simulink subsystem "PvtSubSys_AHBC"  (R2020b)
settings: Solver=VariableStepAuto  StartTime=0.0  StopTime=10.0  RelTol=1e-3
undefined symbols (not defined in the file): P_AHBC_ABS_ENABLE, P_AHBC_DRIVE_DIRECTION_ENABLE, P_AHBC_ESP_ENABLE, P_AHBC_FOG_ENABLE, P_AHBC_FOG_TIME, P_AHBC_HIGHBEAM_ACTIVE_GRACE, P_AHBC_LAT_ACC_ENTER, P_AHBC_LAT_ACC_EXIT, P_AHBC_MAX_ONCOMING_DISTANCE_COUPLE2, P_AHBC_MAX_ONCOMING_DISTANCE_ONE2, P_AHBC_MAX_TAILLIGHT_DISTANCE_COUPLE2, P_AHBC_MAX_TAILLIGHT_DISTANCE_ONE2, P_AHBC_SPEED_SWITCH_HIGH_BEAM_OFF2, P_AHBC_SPEED_SWITCH_HIGH_BEAM_ON2, P_AHBC_TrafficStyle, P_AHBC_TURN_LAMP_ENABLE, P_AHBC_WIPER_ENABLE, P_AHBC_WIPER_TIME, P_AHBC_YAW_RATE_ENTER, P_AHBC_YAW_RATE_EXIT
libraries: simulink x57
(part 2 of 4)

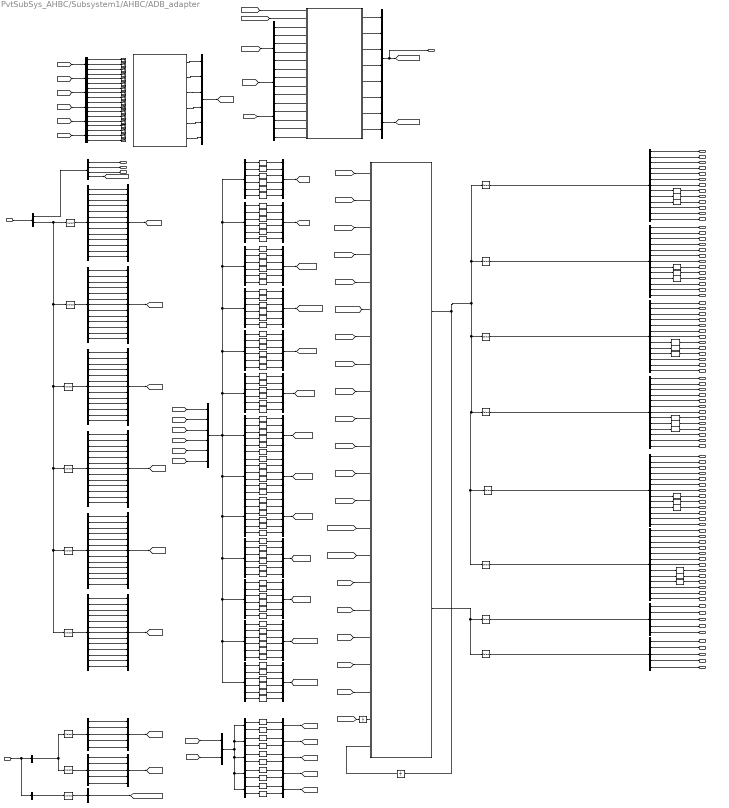
== system PvtSubSys_AHBC/Subsystem1/AHBC/ADB_adapter ==
  EQ4_LSV : Inport  OutDataTypeStr=Bus: EQ4_LSV_BUS
  EQ4_LSR : Inport  Port=2  OutDataTypeStr=Bus: EQ4_LSR_BUS
  Bus Creator{,1..5} (6 alike) : BusCreator  Inputs=13
  Bus Creator{6..20,30} (16 alike) : BusCreator  Inputs=6
  Bus Creator21 : BusCreator  Inputs=5
  Bus Creator22 : BusCreator  Inputs=5
  Bus Creator{23..29} (7 alike) : BusCreator  Inputs=2
  Bus Selector : BusSelector  OutputSignals=EQ4_LSV_HDR,EQ4_LSV_ELEM
  Bus Selector{1..6} (6 alike) : BusSelector  OutputSignals=LSV_ID,LSV_Is_New,LSV_Confidence,LSV_Consecutive_Detection,LSV_Type,LSV_Sub_Type,LSV_CL_Sub_Type,LSV_Distance,LSV_Right_Angle,LSV_Left_Angle,LSV_Top_Angle,LSV_Angular_Velocity_Right,LSV_Angular_Velocity_Left
  Bus Selector10 : BusSelector  OutputSignals=LSV_Running_Mode,LSV_HLB_Decision,LSV_HLB_Reason,LSV_Vehicles_Count
  Bus Selector11 : BusSelector  OutputSignals=EQ4_LSR_HDR
  Bus Selector12 : BusSelector  OutputSignals=LSR_Strong_Reflectors_Count
  Bus Selector13 : BusSelector  OutputSignals=LSV_Elem1.LSV_ID,LSV_Elem2.LSV_ID,LSV_Elem3.LSV_ID,LSV_Elem4.LSV_ID,LSV_Elem5.LSV_ID,LSV_Elem6.LSV_ID
  Bus Selector14 : BusSelector  OutputSignals=LSV_Elem1.LSV_Is_New,LSV_Elem2.LSV_Is_New,LSV_Elem3.LSV_Is_New,LSV_Elem4.LSV_Is_New,LSV_Elem5.LSV_Is_New,LSV_Elem6.LSV_Is_New
  Bus Selector15 : BusSelector  OutputSignals=LSV_Elem1.LSV_Confidence,LSV_Elem2.LSV_Confidence,LSV_Elem3.LSV_Confidence,LSV_Elem4.LSV_Confidence,LSV_Elem5.LSV_Confidence,LSV_Elem6.LSV_Confidence
  Bus Selector16 : BusSelector  OutputSignals=LSV_Elem1.LSV_Consecutive_Detection,LSV_Elem2.LSV_Consecutive_Detection,LSV_Elem3.LSV_Consecutive_Detection,LSV_Elem4.LSV_Consecutive_Detection,LSV_Elem5.LSV_Consecutive_Detection,LSV_Elem6.LSV_Consecutive_Detection
  Bus Selector17 : BusSelector  OutputSignals=LSV_Elem1.LSV_Type,LSV_Elem2.LSV_Type,LSV_Elem3.LSV_Type,LSV_Elem4.LSV_Type,LSV_Elem5.LSV_Type,LSV_Elem6.LSV_Type
  Bus Selector18 : BusSelector  OutputSignals=LSV_Elem1.LSV_Sub_Type,LSV_Elem2.LSV_Sub_Type,LSV_Elem3.LSV_Sub_Type,LSV_Elem4.LSV_Sub_Type,LSV_Elem5.LSV_Sub_Type,LSV_Elem6.LSV_Sub_Type
  Bus Selector19 : BusSelector  OutputSignals=LSV_Elem1.LSV_CL_Sub_Type,LSV_Elem2.LSV_CL_Sub_Type,LSV_Elem3.LSV_CL_Sub_Type,LSV_Elem4.LSV_CL_Sub_Type,LSV_Elem5.LSV_CL_Sub_Type,LSV_Elem6.LSV_CL_Sub_Type
  Bus Selector20 : BusSelector  OutputSignals=LSV_Elem1.LSV_Distance,LSV_Elem2.LSV_Distance,LSV_Elem3.LSV_Distance,LSV_Elem4.LSV_Distance,LSV_Elem5.LSV_Distance,LSV_Elem6.LSV_Distance
  Bus Selector21 : BusSelector  OutputSignals=LSV_Elem1.LSV_Right_Angle,LSV_Elem2.LSV_Right_Angle,LSV_Elem3.LSV_Right_Angle,LSV_Elem4.LSV_Right_Angle,LSV_Elem5.LSV_Right_Angle,LSV_Elem6.LSV_Right_Angle
  Bus Selector22 : BusSelector  OutputSignals=LSV_Elem1.LSV_Left_Angle,LSV_Elem2.LSV_Left_Angle,LSV_Elem3.LSV_Left_Angle,LSV_Elem4.LSV_Left_Angle,LSV_Elem5.LSV_Left_Angle,LSV_Elem6.LSV_Left_Angle
  Bus Selector23 : BusSelector  OutputSignals=LSV_Elem1.LSV_Top_Angle,LSV_Elem2.LSV_Top_Angle,LSV_Elem3.LSV_Top_Angle,LSV_Elem4.LSV_Top_Angle,LSV_Elem5.LSV_Top_Angle,LSV_Elem6.LSV_Top_Angle
  Bus Selector24 : BusSelector  OutputSignals=LSV_Elem1.LSV_Angular_Velocity_Right,LSV_Elem2.LSV_Angular_Velocity_Right,LSV_Elem3.LSV_Angular_Velocity_Right,LSV_Elem4.LSV_Angular_Velocity_Right,LSV_Elem5.LSV_Angular_Velocity_Right,LSV_Elem6.LSV_Angular_Velocity_Right
  Bus Selector25 : BusSelector  OutputSignals=LSV_Elem1.LSV_Angular_Velocity_Left,LSV_Elem2.LSV_Angular_Velocity_Left,LSV_Elem3.LSV_Angular_Velocity_Left,LSV_Elem4.LSV_Angular_Velocity_Left,LSV_Elem5.LSV_Angular_Velocity_Left,LSV_Elem6.LSV_Angular_Velocity_Left
  Bus Selector{26,28..32} (6 alike) : BusSelector  OutputSignals=LSV_ID_Out,LSV_Is_New_Out,LSV_Confidence_Out,LSV_Consecutive_Detection_Out,LSV_Type_Out,LSV_Sub_Type_Out,LSV_CL_Sub_Type_Out,LSV_Distance_Out,LSV_Right_Angle_Out,LSV_Left_Angle_Out,LSV_Top_Angle_Out,LSV_Angular_Velocity_Right_Out,LSV_Angular_Velocity_Left_Out
  Bus Selector27 : BusSelector  OutputSignals=LSV_Distance1,LSV_Distance2,LSV_Distance3,LSV_Distance4,LSV_Distance5,LSV_Distance6
  Bus Selector33 : BusSelector  OutputSignals=LSR_Elem1.LSR_ID,LSR_Elem2.LSR_ID
  Bus Selector34 : BusSelector  OutputSignals=LSR_Elem1.LSR_Distance,LSR_Elem2.LSR_Distance
  Bus Selector35 : BusSelector  OutputSignals=LSR_Elem1.LSR_Right_Angle,LSR_Elem2.LSR_Right_Angle
  Bus Selector36 : BusSelector  OutputSignals=LSR_Elem1.LSR_Left_Angle,LSR_Elem2.LSR_Left_Angle
  Bus Selector37 : BusSelector  OutputSignals=LSR_Elem1.LSR_Top_Angle,LSR_Elem2.LSR_Top_Angle
  Bus Selector38 : BusSelector  OutputSignals=LSR_Distance1,LSR_Distance2
  Bus Selector39 : BusSelector  OutputSignals=LSR_ID_Out,LSR_Distance_Out,LSR_Right_Angle_Out,LSR_Left_Angle_Out,LSR_Top_Angle_Out
  Bus Selector40 : BusSelector  OutputSignals=LSR_ID_Out,LSR_Distance_Out,LSR_Right_Angle_Out,LSR_Left_Angle_Out,LSR_Top_Angle_Out
  Bus Selector{41..46} (6 alike) : BusSelector  OutputSignals=LSV_Left_Angle,LSV_Right_Angle,LSV_Distance
  Bus Selector47 : BusSelector  OutputSignals=Target1_valid,Target2_valid,Target3_valid,Target4_valid,Target5_valid,Target6_valid
  Bus Selector7 : BusSelector  OutputSignals=EQ4_LSR_ELEM
  Bus Selector8 : BusSelector  OutputSignals=LSR_ID,LSR_Distance,LSR_Right_Angle,LSR_Left_Angle,LSR_Top_Angle
  Bus Selector9 : BusSelector  OutputSignals=LSR_ID,LSR_Distance,LSR_Right_Angle,LSR_Left_Angle,LSR_Top_Angle
  MATLAB Function : MATLAB Function  TreatAsAtomicUnit=on
  MATLAB Function1 : MATLAB Function  TreatAsAtomicUnit=on
  MATLAB Function2 : MATLAB Function  TreatAsAtomicUnit=on
  Selector : Selector  InputPortWidth=2  IndexOptions=Index vector (dialog)  Indices=1  OutputSizes=1
  Selector1 : Selector  InputPortWidth=2  IndexOptions=Index vector (dialog)  Indices=2  OutputSizes=1
  Selector10 : Selector  InputPortWidth=2  IndexOptions=Index vector (dialog)  Indices=1  OutputSizes=1
  Selector11 : Selector  InputPortWidth=2  IndexOptions=Index vector (dialog)  Indices=2  OutputSizes=1
  Selector14 : Selector  InputPortWidth=6  IndexOptions=Index vector (dialog)  Indices=2  OutputSizes=1
  Selector15 : Selector  InputPortWidth=6  IndexOptions=Index vector (dialog)  Indices=6  OutputSizes=1
  Selector16 : Selector  InputPortWidth=6  IndexOptions=Index vector (dialog)  Indices=3  OutputSizes=1
  Selector2 : Selector  InputPortWidth=6  IndexOptions=Index vector (dialog)  Indices=1  OutputSizes=1
  Selector23 : Selector  InputPortWidth=6  IndexOptions=Index vector (dialog)  Indices=5  OutputSizes=1
  Selector3 : Selector  InputPortWidth=1  IndexOptions=Index vector (dialog)  Indices=1  OutputSizes=1
  Selector30 : Selector  InputPortWidth=6  IndexOptions=Index vector (dialog)  Indices=4  OutputSizes=1
  Selector4 : Selector  InputPortWidth=6  IndexOptions=Index vector (dialog)  Indices=1  OutputSizes=1
  Selector5 : Selector  InputPortWidth=6  IndexOptions=Index vector (dialog)  Indices=2  OutputSizes=1
  Selector6 : Selector  InputPortWidth=6  IndexOptions=Index vector (dialog)  Indices=3  OutputSizes=1
  Selector7 : Selector  InputPortWidth=6  IndexOptions=Index vector (dialog)  Indices=4  OutputSizes=1
  Selector8 : Selector  InputPortWidth=6  IndexOptions=Index vector (dialog)  Indices=5  OutputSizes=1
  Selector9 : Selector  InputPortWidth=6  IndexOptions=Index vector (dialog)  Indices=6  OutputSizes=1
  Signal Conversion{,1..105} (106 alike) : SignalConversion  OverrideOpt=off
  Terminator{,1..17} (18 alike) : Terminator
  Unit Delay : UnitDelay  SampleTime=-1  HasFrameUpgradeWarning=on
  Unit Delay1 : UnitDelay  SampleTime=-1  HasFrameUpgradeWarning=on
  LSV_Running_Mode : Outport
  LSV_HLB_Decision : Outport  Port=2
  LSV_HLB_Reason : Outport  Port=3
  LSV_ID1 : Outport  Port=4
  LSV_Is_New1 : Outport  Port=5
  LSV_Confidence1 : Outport  Port=6
  LSV_Consecutive_Detection1 : Outport  Port=7
  LSV_Type1 : Outport  Port=8
  LSV_Sub_Type1 : Outport  Port=9
  LSV_CL_Sub_Type1 : Outport  Port=10
  LSV_Distance1 : Outport  Port=11  OutDataTypeStr=uint16
  LSV_Right_Angle1 : Outport  Port=12
  LSV_Left_Angle1 : Outport  Port=13
  LSV_Top_Angle1 : Outport  Port=14
  LSV_Angular_Velocity_Right1 : Outport  Port=15
  LSV_Angular_Velocity_Left1 : Outport  Port=16
  LSV_ID2 : Outport  Port=17
  LSV_Is_New2 : Outport  Port=18
  LSV_Confidence2 : Outport  Port=19
  LSV_Consecutive_Detection2 : Outport  Port=20
  LSV_Type2 : Outport  Port=21
  LSV_Distance2 : Outport  Port=22  OutDataTypeStr=uint16
  LSV_Right_Angle2 : Outport  Port=23
  LSV_Left_Angle2 : Outport  Port=24
  LSV_Top_Angle2 : Outport  Port=25
  LSV_Angular_Velocity_Right2 : Outport  Port=26
  LSV_Angular_Velocity_Left2 : Outport  Port=27
  LSV_Sub_Type2 : Outport  Port=28
  LSV_CL_Sub_Type2 : Outport  Port=29
  LSV_ID3 : Outport  Port=30
  LSV_Is_New3 : Outport  Port=31
  LSV_Confidence3 : Outport  Port=32
  LSV_Consecutive_Detection3 : Outport  Port=33
  LSV_Type3 : Outport  Port=34
  LSV_Sub_Type3 : Outport  Port=35
  LSV_CL_Sub_Type3 : Outport  Port=36
  LSV_Distance3 : Outport  Port=37  OutDataTypeStr=uint16
  LSV_Right_Angle3 : Outport  Port=38
  LSV_Left_Angle3 : Outport  Port=39
  LSV_Top_Angle3 : Outport  Port=40
  LSV_Angular_Velocity_Right3 : Outport  Port=41
  LSV_Angular_Velocity_Left3 : Outport  Port=42
  LSV_ID4 : Outport  Port=43
  LSV_Is_New4 : Outport  Port=44
  LSV_Confidence4 : Outport  Port=45
  LSV_Consecutive_Detection4 : Outport  Port=46
  LSV_Type4 : Outport  Port=47
  LSV_Sub_Type4 : Outport  Port=48
  LSV_CL_Sub_Type4 : Outport  Port=49
  LSV_Distance4 : Outport  Port=50  OutDataTypeStr=uint16
  LSV_Right_Angle4 : Outport  Port=51
  LSV_Left_Angle4 : Outport  Port=52
  LSV_Top_Angle4 : Outport  Port=53
  LSV_Angular_Velocity_Right4 : Outport  Port=54
  LSV_Angular_Velocity_Left4 : Outport  Port=55
  LSV_ID5 : Outport  Port=56
  LSV_Is_New5 : Outport  Port=57
  LSV_Confidence5 : Outport  Port=58
  LSV_Consecutive_Detection5 : Outport  Port=59
  LSV_Type5 : Outport  Port=60
  LSV_Sub_Type5 : Outport  Port=61
  LSV_CL_Sub_Type5 : Outport  Port=62
  LSV_Distance5 : Outport  Port=63  OutDataTypeStr=uint16
  LSV_Right_Angle5 : Outport  Port=64
  LSV_Left_Angle5 : Outport  Port=65
  LSV_Top_Angle5 : Outport  Port=66
  LSV_Angular_Velocity_Right5 : Outport  Port=67
  LSV_Angular_Velocity_Left5 : Outport  Port=68
  LSV_ID6 : Outport  Port=69
  LSV_Is_New6 : Outport  Port=70
  LSV_Confidence6 : Outport  Port=71
  LSV_Consecutive_Detection6 : Outport  Port=72
  LSV_Type6 : Outport  Port=73
  LSV_Sub_Type6 : Outport  Port=74
  LSV_CL_Sub_Type6 : Outport  Port=75
  LSV_Distance6 : Outport  Port=76  OutDataTypeStr=uint16
  LSV_Right_Angle6 : Outport  Port=77
  LSV_Left_Angle6 : Outport  Port=78
  LSV_Top_Angle6 : Outport  Port=79
  LSV_Angular_Velocity_Right6 : Outport  Port=80
  LSV_Angular_Velocity_Left6 : Outport  Port=81
  LSR_ID1 : Outport  Port=82
  LSR_Distance1 : Outport  Port=83  OutDataTypeStr=uint16
  LSR_Right_Angle1 : Outport  Port=84
  LSR_Left_Angle1 : Outport  Port=85
  LSR_Top_Angle1 : Outport  Port=86
  LSR_ID2 : Outport  Port=87
  LSR_Distance2 : Outport  Port=88  OutDataTypeStr=uint16
  LSR_Right_Angle2 : Outport  Port=89
  LSR_Left_Angle2 : Outport  Port=90
  LSR_Top_Angle2 : Outport  Port=91
  LSV_valid_state : Outport  Port=92
  wires:
  Bus Selector46/3 -> Terminator16/1  "<LSV_Distance>"
  Bus Selector46/2 -> Terminator15/1  "<LSV_Right_Angle>"
  Bus Selector46/1 -> Terminator17/1  "<LSV_Left_Angle>"
  Bus Selector45/1 -> Terminator14/1  "<LSV_Left_Angle>"
  Bus Selector45/2 -> Terminator12/1  "<LSV_Right_Angle>"
  Bus Selector45/3 -> Terminator13/1  "<LSV_Distance>"
  Bus Selector44/3 -> Terminator11/1  "<LSV_Distance>"
  Bus Selector44/2 -> Terminator10/1  "<LSV_Right_Angle>"
  Bus Selector44/1 -> Terminator9/1  "<LSV_Left_Angle>"
  Bus Selector43/3 -> Terminator8/1  "<LSV_Distance>"
  Bus Selector43/2 -> Terminator7/1  "<LSV_Right_Angle>"
  Bus Selector43/1 -> Terminator6/1  "<LSV_Left_Angle>"
  Bus Selector42/3 -> Terminator5/1  "<LSV_Distance>"
  Bus Selector42/2 -> Terminator4/1  "<LSV_Right_Angle>"
  Bus Selector42/1 -> Terminator3/1  "<LSV_Left_Angle>"
  Bus Selector41/3 -> Terminator2/1  "<LSV_Distance>"
  Bus Selector41/2 -> Terminator1/1  "<LSV_Right_Angle>"
  Bus Selector41/1 -> Terminator/1  "<LSV_Left_Angle>"
  Unit Delay1/1 -> MATLAB Function1/21(LSV_valid_stateK)
  [LSV_valid_state] -> Unit Delay1/1
  Bus Creator30/1 -> [Target_valid]
  MATLAB Function2/6(Target6_valid) -> Bus Creator30/6
  MATLAB Function2/5(Target5_valid) -> Bus Creator30/5
  MATLAB Function2/4(Target4_valid) -> Bus Creator30/4
  MATLAB Function2/3(Target3_valid) -> Bus Creator30/3
  MATLAB Function2/2(Target2_valid) -> Bus Creator30/2
  MATLAB Function2/1(Target1_valid) -> Bus Creator30/1
  [LSV_Elem6] -> Bus Selector46/1
  [LSV_Elem5] -> Bus Selector45/1
  [LSV_Elem4] -> Bus Selector44/1
  [LSV_Elem3] -> Bus Selector43/1
  [LSV_Elem2] -> Bus Selector42/1
  Signal Conversion14/1 -> LSV_Right_Angle6/1
  Signal Conversion15/1 -> LSV_Left_Angle6/1
  Signal Conversion13/1 -> LSV_Distance6/1
  Signal Conversion104/1 -> LSV_Right_Angle5/1
  Signal Conversion103/1 -> LSV_Distance5/1
  Signal Conversion105/1 -> LSV_Left_Angle5/1
  Signal Conversion101/1 -> LSV_Right_Angle4/1
  Signal Conversion102/1 -> LSV_Left_Angle4/1
  Signal Conversion100/1 -> LSV_Distance4/1
  Signal Conversion99/1 -> LSV_Left_Angle3/1
  Signal Conversion97/1 -> LSV_Distance3/1
  Signal Conversion98/1 -> LSV_Right_Angle3/1
  Signal Conversion16/1 -> LSV_Distance2/1
  Signal Conversion17/1 -> LSV_Right_Angle2/1
  Signal Conversion96/1 -> LSV_Left_Angle2/1
  Signal Conversion12/1 -> LSV_Left_Angle1/1
  Signal Conversion11/1 -> LSV_Right_Angle1/1
  Signal Conversion/1 -> LSV_Distance1/1
  Selector11/1 -> Bus Selector40/1
  Selector10/1 -> Bus Selector39/1
  Bus Selector40/5 -> LSR_Top_Angle2/1  "<LSR_Top_Angle_Out>"
  Bus Selector40/4 -> LSR_Left_Angle2/1  "<LSR_Left_Angle_Out>"
  Bus Selector40/3 -> LSR_Right_Angle2/1  "<LSR_Right_Angle_Out>"
  Bus Selector40/2 -> LSR_Distance2/1  "<LSR_Distance_Out>"
  Bus Selector40/1 -> LSR_ID2/1  "<LSR_ID_Out>"
  Bus Selector39/5 -> LSR_Top_Angle1/1  "<LSR_Top_Angle_Out>"
  Bus Selector39/4 -> LSR_Left_Angle1/1  "<LSR_Left_Angle_Out>"
  Bus Selector39/3 -> LSR_Right_Angle1/1  "<LSR_Right_Angle_Out>"
  Bus Selector39/2 -> LSR_Distance1/1  "<LSR_Distance_Out>"
  Bus Selector39/1 -> LSR_ID1/1  "<LSR_ID_Out>"
  MATLAB Function1/2(LSR_List) -> Selector11/1, Selector10/1
  [LSR_Left_Angle] -> MATLAB Function1/19(LSR_Left_Angle)
  [LSR_Top_Angle] -> MATLAB Function1/20(LSR_Top_Angle)
  [LSR_Right_Angle] -> MATLAB Function1/18(LSR_Right_Angle)
  [LSR_Distance] -> MATLAB Function1/17(LSR_Distance)
  [LSR_ID] -> MATLAB Function1/16(LSR_ID)
  [LSR_valid_state] -> MATLAB Function1/2(LSR_valid_state)
  Bus Creator29/1 -> [LSR_valid_state]  "LSR_valid_state"
  MATLAB Function/7(LSR_valid_state1) -> Bus Creator29/1
  MATLAB Function/8(LSR_valid_state2) -> Bus Creator29/2
  MATLAB Function/6(LSV_valid_state6) -> Bus Creator20/6
  MATLAB Function/5(LSV_valid_state5) -> Bus Creator20/5
  MATLAB Function/4(LSV_valid_state4) -> Bus Creator20/4
  MATLAB Function/3(LSV_valid_state3) -> Bus Creator20/3
  MATLAB Function/2(LSV_valid_state2) -> Bus Creator20/2
  MATLAB Function/1(LSV_valid_state1) -> Bus Creator20/1
  Bus Selector38/2 -> MATLAB Function/10(LSR_Distance2)  "<LSR_Distance2>"
  Bus Selector38/1 -> MATLAB Function/9(LSR_Distance1)  "<LSR_Distance1>"
  [LSR_Distance] -> Bus Selector38/1
  Bus Creator28/1 -> [LSR_Top_Angle]  "LSR_Top_Angle"
  Bus Creator27/1 -> [LSR_Left_Angle]  "LSR_Left_Angle"
  Bus Creator26/1 -> [LSR_Right_Angle]  "LSR_Right_Angle"
  Bus Creator25/1 -> [LSR_Distance]  "LSR_Distance"
  Bus Creator24/1 -> [LSR_ID]  "LSR_ID"
  Signal Conversion10/1 -> Bus Creator28/2  "LSR_Top_Angle2"
  Signal Conversion9/1 -> Bus Creator28/1  "LSR_Top_Angle1"
  Signal Conversion8/1 -> Bus Creator27/2  "LSR_Left_Angle2"
  Signal Conversion7/1 -> Bus Creator27/1  "LSR_Left_Angle1"
  Signal Conversion6/1 -> Bus Creator26/2  "LSR_Right_Angle2"
  Signal Conversion5/1 -> Bus Creator26/1  "LSR_Right_Angle1"
  Signal Conversion4/1 -> Bus Creator25/2  "LSR_Distance2"
  Signal Conversion3/1 -> Bus Creator25/1  "LSR_Distance1"
  Signal Conversion2/1 -> Bus Creator24/2  "LSR_ID2"
  Signal Conversion1/1 -> Bus Creator24/1  "LSR_ID1"
  Bus Selector37/2 -> Signal Conversion10/1  "<LSR_Top_Angle>"
  Bus Selector37/1 -> Signal Conversion9/1  "<LSR_Top_Angle>"
  Bus Selector36/2 -> Signal Conversion8/1  "<LSR_Left_Angle>"
  Bus Selector36/1 -> Signal Conversion7/1  "<LSR_Left_Angle>"
  Bus Selector35/2 -> Signal Conversion6/1  "<LSR_Right_Angle>"
  Bus Selector35/1 -> Signal Conversion5/1  "<LSR_Right_Angle>"
  Bus Selector34/2 -> Signal Conversion4/1  "<LSR_Distance>"
  Bus Selector34/1 -> Signal Conversion3/1  "<LSR_Distance>"
  Bus Selector33/2 -> Signal Conversion2/1  "<LSR_ID>"
  Bus Selector33/1 -> Signal Conversion1/1  "<LSR_ID>"
  Bus Creator23/1 -> Bus Selector35/1, Bus Selector36/1, Bus Selector37/1, Bus Selector33/1, Bus Selector34/1
  [LSR_Elem2] -> Bus Creator23/2
  [LSR_Elem1] -> Bus Creator23/1
  Bus Creator22/1 -> [LSR_Elem2]  "LSR_Elem2"
  Bus Creator21/1 -> [LSR_Elem1]  "LSR_Elem1"
  [LSR_Strong_Reflectors_Count] -> MATLAB Function/2(LSR_Strong_Reflectors_Count)
  Bus Selector12/1 -> [LSR_Strong_Reflectors_Count]  "<LSR_Strong_Reflectors_Count>"
  Bus Selector8/5 -> Bus Creator22/5  "<LSR_Top_Angle>"
  Bus Selector8/4 -> Bus Creator22/4  "<LSR_Left_Angle>"
  Bus Selector8/3 -> Bus Creator22/3  "<LSR_Right_Angle>"
  Bus Selector8/2 -> Bus Creator22/2  "<LSR_Distance>"
  Bus Selector8/1 -> Bus Creator22/1  "<LSR_ID>"
  Bus Selector9/5 -> Bus Creator21/5  "<LSR_Top_Angle>"
  Bus Selector9/4 -> Bus Creator21/4  "<LSR_Left_Angle>"
  Bus Selector9/3 -> Bus Creator21/3  "<LSR_Right_Angle>"
  Bus Selector9/2 -> Bus Creator21/2  "<LSR_Distance>"
  Bus Selector9/1 -> Bus Creator21/1  "<LSR_ID>"
  Bus Selector32/13 -> LSV_Angular_Velocity_Left6/1  "<LSV_Angular_Velocity_Left_Out>"
  Bus Selector32/12 -> LSV_Angular_Velocity_Right6/1  "<LSV_Angular_Velocity_Right_Out>"
  Bus Selector32/11 -> LSV_Top_Angle6/1  "<LSV_Top_Angle_Out>"
  Bus Selector32/10 -> Signal Conversion15/1  "<LSV_Left_Angle_Out>"
  Bus Selector32/9 -> Signal Conversion14/1  "<LSV_Right_Angle_Out>"
  Bus Selector32/8 -> Signal Conversion13/1  "<LSV_Distance_Out>"
  Bus Selector32/7 -> LSV_CL_Sub_Type6/1  "<LSV_CL_Sub_Type_Out>"
  Bus Selector32/6 -> LSV_Sub_Type6/1  "<LSV_Sub_Type_Out>"
  Bus Selector32/5 -> LSV_Type6/1  "<LSV_Type_Out>"
  Bus Selector32/4 -> LSV_Consecutive_Detection6/1  "<LSV_Consecutive_Detection_Out>"
  Bus Selector32/3 -> LSV_Confidence6/1  "<LSV_Confidence_Out>"
  Bus Selector32/2 -> LSV_Is_New6/1  "<LSV_Is_New_Out>"
  Bus Selector32/1 -> LSV_ID6/1  "<LSV_ID_Out>"
  Selector9/1 -> Bus Selector32/1
  Bus Selector31/13 -> LSV_Angular_Velocity_Left5/1  "<LSV_Angular_Velocity_Left_Out>"
  Bus Selector31/12 -> LSV_Angular_Velocity_Right5/1  "<LSV_Angular_Velocity_Right_Out>"
  Bus Selector31/11 -> LSV_Top_Angle5/1  "<LSV_Top_Angle_Out>"
  Bus Selector31/10 -> Signal Conversion105/1  "<LSV_Left_Angle_Out>"
  Bus Selector31/9 -> Signal Conversion104/1  "<LSV_Right_Angle_Out>"
  Bus Selector31/8 -> Signal Conversion103/1  "<LSV_Distance_Out>"
  Bus Selector31/7 -> LSV_CL_Sub_Type5/1  "<LSV_CL_Sub_Type_Out>"
  Bus Selector31/6 -> LSV_Sub_Type5/1  "<LSV_Sub_Type_Out>"
  Bus Selector31/5 -> LSV_Type5/1  "<LSV_Type_Out>"
  Bus Selector31/4 -> LSV_Consecutive_Detection5/1  "<LSV_Consecutive_Detection_Out>"
  Bus Selector31/3 -> LSV_Confidence5/1  "<LSV_Confidence_Out>"
  Bus Selector31/2 -> LSV_Is_New5/1  "<LSV_Is_New_Out>"
  Bus Selector31/1 -> LSV_ID5/1  "<LSV_ID_Out>"
  Selector8/1 -> Bus Selector31/1
  Bus Selector30/13 -> LSV_Angular_Velocity_Left4/1  "<LSV_Angular_Velocity_Left_Out>"
  Bus Selector30/12 -> LSV_Angular_Velocity_Right4/1  "<LSV_Angular_Velocity_Right_Out>"
  Bus Selector30/11 -> LSV_Top_Angle4/1  "<LSV_Top_Angle_Out>"
  Bus Selector30/10 -> Signal Conversion102/1  "<LSV_Left_Angle_Out>"
  Bus Selector30/9 -> Signal Conversion101/1  "<LSV_Right_Angle_Out>"
  Bus Selector30/8 -> Signal Conversion100/1  "<LSV_Distance_Out>"
  Bus Selector30/7 -> LSV_CL_Sub_Type4/1  "<LSV_CL_Sub_Type_Out>"
  Bus Selector30/6 -> LSV_Sub_Type4/1  "<LSV_Sub_Type_Out>"
  Bus Selector30/5 -> LSV_Type4/1  "<LSV_Type_Out>"
  Bus Selector30/4 -> LSV_Consecutive_Detection4/1  "<LSV_Consecutive_Detection_Out>"
  Bus Selector30/3 -> LSV_Confidence4/1  "<LSV_Confidence_Out>"
  Bus Selector30/2 -> LSV_Is_New4/1  "<LSV_Is_New_Out>"
  Bus Selector30/1 -> LSV_ID4/1  "<LSV_ID_Out>"
  Selector7/1 -> Bus Selector30/1
  Selector6/1 -> Bus Selector29/1
  Bus Selector29/13 -> LSV_Angular_Velocity_Left3/1  "<LSV_Angular_Velocity_Left_Out>"
  Bus Selector29/12 -> LSV_Angular_Velocity_Right3/1  "<LSV_Angular_Velocity_Right_Out>"
  Bus Selector29/11 -> LSV_Top_Angle3/1  "<LSV_Top_Angle_Out>"
  Bus Selector29/10 -> Signal Conversion99/1  "<LSV_Left_Angle_Out>"
  Bus Selector29/9 -> Signal Conversion98/1  "<LSV_Right_Angle_Out>"
  Bus Selector29/8 -> Signal Conversion97/1  "<LSV_Distance_Out>"
  Bus Selector29/7 -> LSV_CL_Sub_Type3/1  "<LSV_CL_Sub_Type_Out>"
  Bus Selector29/6 -> LSV_Sub_Type3/1  "<LSV_Sub_Type_Out>"
  Bus Selector29/5 -> LSV_Type3/1  "<LSV_Type_Out>"
  Bus Selector29/4 -> LSV_Consecutive_Detection3/1  "<LSV_Consecutive_Detection_Out>"
  Bus Selector29/3 -> LSV_Confidence3/1  "<LSV_Confidence_Out>"
  Bus Selector29/2 -> LSV_Is_New3/1  "<LSV_Is_New_Out>"
  Bus Selector29/1 -> LSV_ID3/1  "<LSV_ID_Out>"
  Selector5/1 -> Bus Selector28/1
  Bus Selector28/13 -> LSV_Angular_Velocity_Left2/1  "<LSV_Angular_Velocity_Left_Out>"
  Bus Selector28/12 -> LSV_Angular_Velocity_Right2/1  "<LSV_Angular_Velocity_Right_Out>"
  Bus Selector28/11 -> LSV_Top_Angle2/1  "<LSV_Top_Angle_Out>"
  Bus Selector28/10 -> Signal Conversion96/1  "<LSV_Left_Angle_Out>"
  Bus Selector28/9 -> Signal Conversion17/1  "<LSV_Right_Angle_Out>"
  Bus Selector28/8 -> Signal Conversion16/1  "<LSV_Distance_Out>"
  Bus Selector28/7 -> LSV_CL_Sub_Type2/1  "<LSV_CL_Sub_Type_Out>"
  Bus Selector28/6 -> LSV_Sub_Type2/1  "<LSV_Sub_Type_Out>"
  Bus Selector28/5 -> LSV_Type2/1  "<LSV_Type_Out>"
  Bus Selector28/4 -> LSV_Consecutive_Detection2/1  "<LSV_Consecutive_Detection_Out>"
  Bus Selector28/3 -> LSV_Confidence2/1  "<LSV_Confidence_Out>"
  Bus Selector28/2 -> LSV_Is_New2/1  "<LSV_Is_New_Out>"
  Bus Selector28/1 -> LSV_ID2/1  "<LSV_ID_Out>"
  Bus Selector26/13 -> LSV_Angular_Velocity_Left1/1  "<LSV_Angular_Velocity_Left_Out>"
  Bus Selector26/12 -> LSV_Angular_Velocity_Right1/1  "<LSV_Angular_Velocity_Right_Out>"
  Bus Selector26/11 -> LSV_Top_Angle1/1  "<LSV_Top_Angle_Out>"
  Bus Selector26/10 -> Signal Conversion12/1  "<LSV_Left_Angle_Out>"
  Bus Selector26/9 -> Signal Conversion11/1  "<LSV_Right_Angle_Out>"
  Bus Selector26/8 -> Signal Conversion/1  "<LSV_Distance_Out>"
  Selector4/1 -> Bus Selector26/1
  MATLAB Function1/1(LSV_List) -> Unit Delay/1, Selector8/1, Selector9/1, Selector7/1, Selector6/1, Selector5/1, Selector4/1
  Bus Selector10/3 -> LSV_HLB_Reason/1  "<LSV_HLB_Reason>"
  Bus Selector10/2 -> LSV_HLB_Decision/1  "<LSV_HLB_Decision>"
  Bus Selector10/1 -> LSV_Running_Mode/1  "<LSV_Running_Mode>"
  [LSV_valid_state] -> MATLAB Function1/1(LSV_valid_state)
  Bus Creator20/1 -> [LSV_valid_state], LSV_valid_state/1  "LSV_valid_state"
  Bus Selector27/6 -> MATLAB Function/8(LSV_Distance6)  "<LSV_Distance6>"
  Bus Selector27/5 -> MATLAB Function/7(LSV_Distance5)  "<LSV_Distance5>"
  Bus Selector27/4 -> MATLAB Function/6(LSV_Distance4)  "<LSV_Distance4>"
  Bus Selector27/3 -> MATLAB Function/5(LSV_Distance3)  "<LSV_Distance3>"
  Bus Selector27/2 -> MATLAB Function/4(LSV_Distance2)  "<LSV_Distance2>"
  Bus Selector27/1 -> MATLAB Function/3(LSV_Distance1)  "<LSV_Distance1>"
  [LSV_Distance] -> Bus Selector27/1
  [LSV_Top_Angle] -> MATLAB Function1/13(LSV_Top_Angle)
  [LSV_Left_Angle] -> MATLAB Function1/12(LSV_Left_Angle)
  [LSV_Angular_Velocity_Right] -> MATLAB Function1/14(LSV_Angular_Velocity_Right)
  [LSV_Angular_Velocity_Left] -> MATLAB Function1/15(LSV_Angular_Velocity_Left)
  [LSV_Right_Angle] -> MATLAB Function1/11(LSV_Right_Angle)
  [LSV_Distance] -> MATLAB Function1/10(LSV_Distance)
  [LSV_CL_Sub_Type] -> MATLAB Function1/9(LSV_CL_Sub_Type)
  [LSV_Sub_Type] -> MATLAB Function1/8(LSV_Sub_Type)
  [LSV_Type] -> MATLAB Function1/7(LSV_Type)
  [LSV_Consecutive_Detection] -> MATLAB Function1/6(LSV_Consecutive_Detection)
  [LSV_Confidence] -> MATLAB Function1/5(LSV_Confidence)
  [LSV_Is_New] -> MATLAB Function1/4(LSV_Is_New)
  [LSV_ID] -> MATLAB Function1/3(LSV_ID)
  Bus Creator19/1 -> [LSV_Angular_Velocity_Left]  "LSV_Angular_Velocity_Left"
  Bus Creator18/1 -> [LSV_Angular_Velocity_Right]  "LSV_Angular_Velocity_Right"
  Bus Creator17/1 -> [LSV_Top_Angle]  "LSV_Top_Angle"
  Bus Creator16/1 -> [LSV_Left_Angle]  "LSV_Left_Angle"
  Bus Creator15/1 -> [LSV_Right_Angle]  "LSV_Right_Angle"
  Bus Creator14/1 -> [LSV_Distance]  "LSV_Distance"
  Bus Creator13/1 -> [LSV_CL_Sub_Type]  "LSV_CL_Sub_Type"
  Bus Creator12/1 -> [LSV_Sub_Type]  "LSV_Sub_Type"
  Bus Creator11/1 -> [LSV_Type]  "LSV_Type"
  Bus Creator10/1 -> [LSV_Consecutive_Detection]  "LSV_Consecutive_Detection"
  Bus Creator9/1 -> [LSV_Confidence]  "LSV_Confidence"
  Bus Creator8/1 -> [LSV_Is_New]  "LSV_Is_New"
  Bus Creator7/1 -> [LSV_ID]  "LSV_ID"
  Bus Selector25/6 -> Signal Conversion95/1  "<LSV_Angular_Velocity_Left>"
  Bus Selector25/5 -> Signal Conversion94/1  "<LSV_Angular_Velocity_Left>"
  Bus Selector25/4 -> Signal Conversion93/1  "<LSV_Angular_Velocity_Left>"
  Bus Selector25/3 -> Signal Conversion92/1  "<LSV_Angular_Velocity_Left>"
  Bus Selector25/2 -> Signal Conversion91/1  "<LSV_Angular_Velocity_Left>"
  Bus Selector25/1 -> Signal Conversion90/1  "<LSV_Angular_Velocity_Left>"
  Signal Conversion90/1 -> Bus Creator19/1  "LSV_Angular_Velocity_Left1"
  Signal Conversion91/1 -> Bus Creator19/2  "LSV_Angular_Velocity_Left2"
  Signal Conversion92/1 -> Bus Creator19/3  "LSV_Angular_Velocity_Left3"
  Signal Conversion93/1 -> Bus Creator19/4  "LSV_Angular_Velocity_Left4"
  Signal Conversion94/1 -> Bus Creator19/5  "LSV_Angular_Velocity_Left5"
  Signal Conversion95/1 -> Bus Creator19/6  "LSV_Angular_Velocity_Left6"
  Bus Selector24/6 -> Signal Conversion89/1  "<LSV_Angular_Velocity_Right>"
  Bus Selector24/5 -> Signal Conversion88/1  "<LSV_Angular_Velocity_Right>"
  Bus Selector24/4 -> Signal Conversion87/1  "<LSV_Angular_Velocity_Right>"
  Bus Selector24/3 -> Signal Conversion86/1  "<LSV_Angular_Velocity_Right>"
  Bus Selector24/2 -> Signal Conversion85/1  "<LSV_Angular_Velocity_Right>"
  Bus Selector24/1 -> Signal Conversion84/1  "<LSV_Angular_Velocity_Right>"
  Signal Conversion89/1 -> Bus Creator18/6  "LSV_Angular_Velocity_Right6"
  Signal Conversion88/1 -> Bus Creator18/5  "LSV_Angular_Velocity_Right5"
  Signal Conversion87/1 -> Bus Creator18/4  "LSV_Angular_Velocity_Right4"
  Signal Conversion86/1 -> Bus Creator18/3  "LSV_Angular_Velocity_Right3"
  Signal Conversion85/1 -> Bus Creator18/2  "LSV_Angular_Velocity_Right2"
  Signal Conversion84/1 -> Bus Creator18/1  "LSV_Angular_Velocity_Right1"
  Bus Selector23/6 -> Signal Conversion83/1  "<LSV_Top_Angle>"
  Bus Selector23/5 -> Signal Conversion82/1  "<LSV_Top_Angle>"
  Bus Selector23/4 -> Signal Conversion81/1  "<LSV_Top_Angle>"
  Bus Selector23/3 -> Signal Conversion80/1  "<LSV_Top_Angle>"
  Bus Selector23/2 -> Signal Conversion79/1  "<LSV_Top_Angle>"
  Bus Selector23/1 -> Signal Conversion78/1  "<LSV_Top_Angle>"
  Signal Conversion78/1 -> Bus Creator17/1  "LSV_Top_Angle1"
  Signal Conversion79/1 -> Bus Creator17/2  "LSV_Top_Angle2"
  Signal Conversion80/1 -> Bus Creator17/3  "LSV_Top_Angle3"
  Signal Conversion81/1 -> Bus Creator17/4  "LSV_Top_Angle4"
  Signal Conversion82/1 -> Bus Creator17/5  "LSV_Top_Angle5"
  Signal Conversion83/1 -> Bus Creator17/6  "LSV_Top_Angle6"
  Bus Selector22/6 -> Signal Conversion77/1  "<LSV_Left_Angle>"
  Bus Selector22/5 -> Signal Conversion76/1  "<LSV_Left_Angle>"
  Bus Selector22/4 -> Signal Conversion75/1  "<LSV_Left_Angle>"
  Bus Selector22/3 -> Signal Conversion74/1  "<LSV_Left_Angle>"
  Bus Selector22/2 -> Signal Conversion73/1  "<LSV_Left_Angle>"
  Bus Selector22/1 -> Signal Conversion72/1  "<LSV_Left_Angle>"
  Signal Conversion77/1 -> Bus Creator16/6  "LSV_Left_Angle6"
  Signal Conversion76/1 -> Bus Creator16/5  "LSV_Left_Angle5"
  Signal Conversion75/1 -> Bus Creator16/4  "LSV_Left_Angle4"
  Signal Conversion74/1 -> Bus Creator16/3  "LSV_Left_Angle3"
  Signal Conversion73/1 -> Bus Creator16/2  "LSV_Left_Angle2"
  Signal Conversion72/1 -> Bus Creator16/1  "LSV_Left_Angle1"
  Bus Selector21/6 -> Signal Conversion71/1  "<LSV_Right_Angle>"
  Bus Selector21/5 -> Signal Conversion70/1  "<LSV_Right_Angle>"
  Bus Selector21/4 -> Signal Conversion69/1  "<LSV_Right_Angle>"
  Bus Selector21/3 -> Signal Conversion68/1  "<LSV_Right_Angle>"
  Bus Selector21/2 -> Signal Conversion67/1  "<LSV_Right_Angle>"
  Bus Selector21/1 -> Signal Conversion66/1  "<LSV_Right_Angle>"
  Bus Selector20/6 -> Signal Conversion65/1  "<LSV_Distance>"
  Bus Selector20/5 -> Signal Conversion64/1  "<LSV_Distance>"
  Bus Selector20/4 -> Signal Conversion63/1  "<LSV_Distance>"
  Bus Selector20/3 -> Signal Conversion62/1  "<LSV_Distance>"
  Bus Selector20/2 -> Signal Conversion61/1  "<LSV_Distance>"
  Bus Selector20/1 -> Signal Conversion60/1  "<LSV_Distance>"
  Signal Conversion66/1 -> Bus Creator15/1  "LSV_Right_Angle1"
  Signal Conversion67/1 -> Bus Creator15/2  "LSV_Right_Angle2"
  Signal Conversion68/1 -> Bus Creator15/3  "LSV_Right_Angle3"
  Signal Conversion69/1 -> Bus Creator15/4  "LSV_Right_Angle4"
  Signal Conversion70/1 -> Bus Creator15/5  "LSV_Right_Angle5"
  Signal Conversion71/1 -> Bus Creator15/6  "LSV_Right_Angle6"
  Signal Conversion65/1 -> Bus Creator14/6  "LSV_Distance6"
  Signal Conversion64/1 -> Bus Creator14/5  "LSV_Distance5"
  Signal Conversion63/1 -> Bus Creator14/4  "LSV_Distance4"
  Signal Conversion62/1 -> Bus Creator14/3  "LSV_Distance3"
  Signal Conversion61/1 -> Bus Creator14/2  "LSV_Distance2"
  Signal Conversion60/1 -> Bus Creator14/1  "LSV_Distance1"
  Signal Conversion54/1 -> Bus Creator13/1  "LSV_CL_Sub_Type1"
  Signal Conversion55/1 -> Bus Creator13/2  "LSV_CL_Sub_Type2"
  Signal Conversion56/1 -> Bus Creator13/3  "LSV_CL_Sub_Type3"
  Signal Conversion57/1 -> Bus Creator13/4  "LSV_CL_Sub_Type4"
  Signal Conversion58/1 -> Bus Creator13/5  "LSV_CL_Sub_Type5"
  Signal Conversion59/1 -> Bus Creator13/6  "LSV_CL_Sub_Type6"
  Bus Selector19/1 -> Signal Conversion54/1  "<LSV_CL_Sub_Type>"
  Bus Selector19/2 -> Signal Conversion55/1  "<LSV_CL_Sub_Type>"
  Bus Selector19/3 -> Signal Conversion56/1  "<LSV_CL_Sub_Type>"
  Bus Selector19/4 -> Signal Conversion57/1  "<LSV_CL_Sub_Type>"
  Bus Selector19/5 -> Signal Conversion58/1  "<LSV_CL_Sub_Type>"
  Bus Selector19/6 -> Signal Conversion59/1  "<LSV_CL_Sub_Type>"
  Bus Selector18/6 -> Signal Conversion53/1  "<LSV_Sub_Type>"
  Bus Selector18/5 -> Signal Conversion52/1  "<LSV_Sub_Type>"
  Bus Selector18/4 -> Signal Conversion51/1  "<LSV_Sub_Type>"
  Bus Selector18/3 -> Signal Conversion50/1  "<LSV_Sub_Type>"
  Bus Selector18/2 -> Signal Conversion49/1  "<LSV_Sub_Type>"
  Bus Selector18/1 -> Signal Conversion48/1  "<LSV_Sub_Type>"
  Signal Conversion53/1 -> Bus Creator12/6  "LSV_Sub_Type6"
  Signal Conversion52/1 -> Bus Creator12/5  "LSV_Sub_Type5"
  Signal Conversion51/1 -> Bus Creator12/4  "LSV_Sub_Type4"
  Signal Conversion50/1 -> Bus Creator12/3  "LSV_Sub_Type3"
  Signal Conversion49/1 -> Bus Creator12/2  "LSV_Sub_Type2"
  Signal Conversion48/1 -> Bus Creator12/1  "LSV_Sub_Type1"
  Bus Selector17/6 -> Signal Conversion47/1  "<LSV_Type>"
  Bus Selector17/5 -> Signal Conversion46/1  "<LSV_Type>"
  Bus Selector17/4 -> Signal Conversion45/1  "<LSV_Type>"
  Bus Selector17/3 -> Signal Conversion44/1  "<LSV_Type>"
  Bus Selector17/2 -> Signal Conversion43/1  "<LSV_Type>"
  Bus Selector17/1 -> Signal Conversion42/1  "<LSV_Type>"
  Signal Conversion42/1 -> Bus Creator11/1  "LSV_Type1"
  Signal Conversion43/1 -> Bus Creator11/2  "LSV_Type2"
  Signal Conversion44/1 -> Bus Creator11/3  "LSV_Type3"
  Signal Conversion45/1 -> Bus Creator11/4  "LSV_Type4"
  Signal Conversion46/1 -> Bus Creator11/5  "LSV_Type5"
  Signal Conversion47/1 -> Bus Creator11/6  "LSV_Type6"
  Bus Selector16/6 -> Signal Conversion41/1  "<LSV_Consecutive_Detection>"
  Bus Selector16/5 -> Signal Conversion40/1  "<LSV_Consecutive_Detection>"
  Bus Selector16/4 -> Signal Conversion39/1  "<LSV_Consecutive_Detection>"
  Bus Selector16/3 -> Signal Conversion38/1  "<LSV_Consecutive_Detection>"
  Bus Selector16/2 -> Signal Conversion37/1  "<LSV_Consecutive_Detection>"
  Bus Selector16/1 -> Signal Conversion36/1  "<LSV_Consecutive_Detection>"
  Signal Conversion36/1 -> Bus Creator10/1  "LSV_Consecutive_Detection1"
  Signal Conversion37/1 -> Bus Creator10/2  "LSV_Consecutive_Detection2"
  Signal Conversion38/1 -> Bus Creator10/3  "LSV_Consecutive_Detection3"
  Signal Conversion39/1 -> Bus Creator10/4  "LSV_Consecutive_Detection4"
  Signal Conversion40/1 -> Bus Creator10/5  "LSV_Consecutive_Detection5"
  Signal Conversion41/1 -> Bus Creator10/6  "LSV_Consecutive_Detection6"
  Signal Conversion35/1 -> Bus Creator9/6  "LSV_Confidence6"
  Signal Conversion34/1 -> Bus Creator9/5  "LSV_Confidence5"
  Signal Conversion33/1 -> Bus Creator9/4  "LSV_Confidence4"
  Signal Conversion32/1 -> Bus Creator9/3  "LSV_Confidence3"
  Signal Conversion31/1 -> Bus Creator9/2  "LSV_Confidence2"
  Signal Conversion30/1 -> Bus Creator9/1  "LSV_Confidence1"
  Bus Selector15/1 -> Signal Conversion30/1  "<LSV_Confidence>"
  Bus Selector15/2 -> Signal Conversion31/1  "<LSV_Confidence>"
  Bus Selector15/3 -> Signal Conversion32/1  "<LSV_Confidence>"
  Bus Selector15/4 -> Signal Conversion33/1  "<LSV_Confidence>"
  Bus Selector15/5 -> Signal Conversion34/1  "<LSV_Confidence>"
  Bus Selector15/6 -> Signal Conversion35/1  "<LSV_Confidence>"
  Bus Selector14/6 -> Signal Conversion29/1  "<LSV_Is_New>"
  Bus Selector14/5 -> Signal Conversion28/1  "<LSV_Is_New>"
  Bus Selector14/4 -> Signal Conversion27/1  "<LSV_Is_New>"
  Bus Selector14/3 -> Signal Conversion26/1  "<LSV_Is_New>"
  Bus Selector14/2 -> Signal Conversion25/1  "<LSV_Is_New>"
  Bus Selector14/1 -> Signal Conversion24/1  "<LSV_Is_New>"
  Signal Conversion24/1 -> Bus Creator8/1  "LSV_Is_New1"
  Signal Conversion25/1 -> Bus Creator8/2  "LSV_Is_New2"
  Signal Conversion26/1 -> Bus Creator8/3  "LSV_Is_New3"
  Signal Conversion27/1 -> Bus Creator8/4  "LSV_Is_New4"
  Signal Conversion28/1 -> Bus Creator8/5  "LSV_Is_New5"
  Signal Conversion29/1 -> Bus Creator8/6  "LSV_Is_New6"
  Signal Conversion23/1 -> Bus Creator7/6  "LSV_ID6"
  Signal Conversion22/1 -> Bus Creator7/5  "LSV_ID5"
  Signal Conversion21/1 -> Bus Creator7/4  "LSV_ID4"
  Signal Conversion20/1 -> Bus Creator7/3  "LSV_ID3"
  Signal Conversion19/1 -> Bus Creator7/2  "LSV_ID2"
  Signal Conversion18/1 -> Bus Creator7/1  "LSV_ID1"
  Bus Selector13/6 -> Signal Conversion23/1  "<LSV_ID>"
  Bus Selector13/5 -> Signal Conversion22/1  "<LSV_ID>"
  Bus Selector13/4 -> Signal Conversion21/1  "<LSV_ID>"
  Bus Selector13/3 -> Signal Conversion20/1  "<LSV_ID>"
  Bus Selector13/2 -> Signal Conversion19/1  "<LSV_ID>"
  Bus Selector13/1 -> Signal Conversion18/1  "<LSV_ID>"
  Bus Creator6/1 -> Bus Selector19/1, Bus Selector20/1, Bus Selector21/1, Bus Selector22/1, Bus Selector23/1, Bus Selector24/1, Bus Selector25/1, Bus Selector18/1, Bus Selector17/1, Bus Selector16/1, Bus Selector15/1, Bus Selector14/1, Bus Selector13/1
  [LSV_Elem6] -> Bus Creator6/6
  [LSV_Elem5] -> Bus Creator6/5
  [LSV_Elem4] -> Bus Creator6/4
  [LSV_Elem3] -> Bus Creator6/3
  [LSV_Elem2] -> Bus Creator6/2
  [LSV_Elem1] -> Bus Creator6/1
  Bus Creator5/1 -> [LSV_Elem6]  "LSV_Elem6"
  Bus Creator4/1 -> [LSV_Elem5]  "LSV_Elem5"
  Bus Creator3/1 -> [LSV_Elem4]  "LSV_Elem4"
  Bus Creator2/1 -> [LSV_Elem3]  "LSV_Elem3"
  Bus Creator1/1 -> [LSV_Elem2]  "LSV_Elem2"
  Bus Creator/1 -> [LSV_Elem1]  "LSV_Elem1"
  Bus Selector6/13 -> Bus Creator5/13  "<LSV_Angular_Velocity_Left>"
  Bus Selector6/12 -> Bus Creator5/12  "<LSV_Angular_Velocity_Right>"
  Bus Selector6/11 -> Bus Creator5/11  "<LSV_Top_Angle>"
  Bus Selector6/10 -> Bus Creator5/10  "<LSV_Left_Angle>"
  Bus Selector6/9 -> Bus Creator5/9  "<LSV_Right_Angle>"
  Bus Selector6/8 -> Bus Creator5/8  "<LSV_Distance>"
  Bus Selector6/7 -> Bus Creator5/7  "<LSV_CL_Sub_Type>"
  Bus Selector6/6 -> Bus Creator5/6  "<LSV_Sub_Type>"
  Bus Selector6/5 -> Bus Creator5/5  "<LSV_Type>"
  Bus Selector6/4 -> Bus Creator5/4  "<LSV_Consecutive_Detection>"
  Bus Selector6/3 -> Bus Creator5/3  "<LSV_Confidence>"
  Bus Selector6/2 -> Bus Creator5/2  "<LSV_Is_New>"
  Bus Selector6/1 -> Bus Creator5/1  "<LSV_ID>"
  Bus Selector5/13 -> Bus Creator4/13  "<LSV_Angular_Velocity_Left>"
  Bus Selector5/12 -> Bus Creator4/12  "<LSV_Angular_Velocity_Right>"
  Bus Selector5/11 -> Bus Creator4/11  "<LSV_Top_Angle>"
  Bus Selector5/10 -> Bus Creator4/10  "<LSV_Left_Angle>"
  Bus Selector5/9 -> Bus Creator4/9  "<LSV_Right_Angle>"
  Bus Selector5/8 -> Bus Creator4/8  "<LSV_Distance>"
  Bus Selector5/7 -> Bus Creator4/7  "<LSV_CL_Sub_Type>"
  Bus Selector5/6 -> Bus Creator4/6  "<LSV_Sub_Type>"
  Bus Selector5/5 -> Bus Creator4/5  "<LSV_Type>"
  Bus Selector5/4 -> Bus Creator4/4  "<LSV_Consecutive_Detection>"
  Bus Selector5/3 -> Bus Creator4/3  "<LSV_Confidence>"
  Bus Selector5/2 -> Bus Creator4/2  "<LSV_Is_New>"
  Bus Selector5/1 -> Bus Creator4/1  "<LSV_ID>"
  Bus Selector4/13 -> Bus Creator3/13  "<LSV_Angular_Velocity_Left>"
  Bus Selector4/12 -> Bus Creator3/12  "<LSV_Angular_Velocity_Right>"
  Bus Selector4/11 -> Bus Creator3/11  "<LSV_Top_Angle>"
  Bus Selector4/10 -> Bus Creator3/10  "<LSV_Left_Angle>"
  Bus Selector4/9 -> Bus Creator3/9  "<LSV_Right_Angle>"
  Bus Selector4/8 -> Bus Creator3/8  "<LSV_Distance>"
  Bus Selector4/7 -> Bus Creator3/7  "<LSV_CL_Sub_Type>"
  Bus Selector4/6 -> Bus Creator3/6  "<LSV_Sub_Type>"
  Bus Selector4/5 -> Bus Creator3/5  "<LSV_Type>"
  Bus Selector4/4 -> Bus Creator3/4  "<LSV_Consecutive_Detection>"
  Bus Selector4/3 -> Bus Creator3/3  "<LSV_Confidence>"
  Bus Selector4/2 -> Bus Creator3/2  "<LSV_Is_New>"
  Bus Selector4/1 -> Bus Creator3/1  "<LSV_ID>"
  Bus Selector3/13 -> Bus Creator2/13  "<LSV_Angular_Velocity_Left>"
  Bus Selector3/12 -> Bus Creator2/12  "<LSV_Angular_Velocity_Right>"
  Bus Selector3/11 -> Bus Creator2/11  "<LSV_Top_Angle>"
  Bus Selector3/10 -> Bus Creator2/10  "<LSV_Left_Angle>"
  Bus Selector3/9 -> Bus Creator2/9  "<LSV_Right_Angle>"
  Bus Selector3/8 -> Bus Creator2/8  "<LSV_Distance>"
  Bus Selector3/7 -> Bus Creator2/7  "<LSV_CL_Sub_Type>"
  Bus Selector3/6 -> Bus Creator2/6  "<LSV_Sub_Type>"
  Bus Selector3/5 -> Bus Creator2/5  "<LSV_Type>"
  Bus Selector3/4 -> Bus Creator2/4  "<LSV_Consecutive_Detection>"
  Bus Selector3/3 -> Bus Creator2/3  "<LSV_Confidence>"
  Bus Selector3/2 -> Bus Creator2/2  "<LSV_Is_New>"
  Bus Selector3/1 -> Bus Creator2/1  "<LSV_ID>"
  Bus Selector1/13 -> Bus Creator1/13  "<LSV_Angular_Velocity_Left>"
  Bus Selector1/12 -> Bus Creator1/12  "<LSV_Angular_Velocity_Right>"
  Bus Selector1/11 -> Bus Creator1/11  "<LSV_Top_Angle>"
  Bus Selector1/10 -> Bus Creator1/10  "<LSV_Left_Angle>"
  Bus Selector1/9 -> Bus Creator1/9  "<LSV_Right_Angle>"
  Bus Selector1/8 -> Bus Creator1/8  "<LSV_Distance>"
  Bus Selector1/7 -> Bus Creator1/7  "<LSV_CL_Sub_Type>"
  Bus Selector1/6 -> Bus Creator1/6  "<LSV_Sub_Type>"
  Bus Selector1/5 -> Bus Creator1/5  "<LSV_Type>"
  Bus Selector1/4 -> Bus Creator1/4  "<LSV_Consecutive_Detection>"
  Bus Selector1/3 -> Bus Creator1/3  "<LSV_Confidence>"
  Bus Selector1/2 -> Bus Creator1/2  "<LSV_Is_New>"
  Bus Selector1/1 -> Bus Creator1/1  "<LSV_ID>"
  Bus Selector2/13 -> Bus Creator/13  "<LSV_Angular_Velocity_Left>"
  Bus Selector2/12 -> Bus Creator/12  "<LSV_Angular_Velocity_Right>"
  Bus Selector2/11 -> Bus Creator/11  "<LSV_Top_Angle>"
  Bus Selector2/10 -> Bus Creator/10  "<LSV_Left_Angle>"
  Bus Selector2/9 -> Bus Creator/9  "<LSV_Right_Angle>"
  Bus Selector2/8 -> Bus Creator/8  "<LSV_Distance>"
  Bus Selector2/7 -> Bus Creator/7  "<LSV_CL_Sub_Type>"
  Bus Selector2/6 -> Bus Creator/6  "<LSV_Sub_Type>"
  Bus Selector2/5 -> Bus Creator/5  "<LSV_Type>"
  Bus Selector2/4 -> Bus Creator/4  "<LSV_Consecutive_Detection>"
  Bus Selector2/3 -> Bus Creator/3  "<LSV_Confidence>"
  Bus Selector2/2 -> Bus Creator/2  "<LSV_Is_New>"
  Bus Selector2/1 -> Bus Creator/1  "<LSV_ID>"
  Bus Selector26/7 -> LSV_CL_Sub_Type1/1  "<LSV_CL_Sub_Type_Out>"
  Bus Selector26/6 -> LSV_Sub_Type1/1  "<LSV_Sub_Type_Out>"
  Bus Selector26/2 -> LSV_Is_New1/1  "<LSV_Is_New_Out>"
  Bus Selector26/5 -> LSV_Type1/1  "<LSV_Type_Out>"
  Bus Selector26/4 -> LSV_Consecutive_Detection1/1  "<LSV_Consecutive_Detection_Out>"
  Bus Selector26/3 -> LSV_Confidence1/1  "<LSV_Confidence_Out>"
  Bus Selector26/1 -> LSV_ID1/1  "<LSV_ID_Out>"
  Selector3/1 -> Bus Selector12/1
  Bus Selector11/1 -> Selector3/1  "<EQ4_LSR_HDR>"
  Selector1/1 -> Bus Selector8/1
  Bus Selector7/1 -> Selector/1, Selector1/1  "<EQ4_LSR_ELEM>"
  Selector/1 -> Bus Selector9/1
  Selector15/1 -> Bus Selector6/1
  Selector23/1 -> Bus Selector5/1
  Selector30/1 -> Bus Selector4/1
  Selector16/1 -> Bus Selector3/1
  Selector14/1 -> Bus Selector1/1
  EQ4_LSR/1 -> Bus Selector7/1, Bus Selector11/1
  Bus Selector/1 -> Bus Selector10/1  "<EQ4_LSV_HDR>"
  EQ4_LSV/1 -> Bus Selector/1
  Bus Selector/2 -> Selector2/1, Selector14/1, Selector16/1, Selector30/1, Selector23/1, Selector15/1  "<EQ4_LSV_ELEM>"
  Selector2/1 -> Bus Selector2/1
  Bus Selector10/4 -> [LSV_Vehicles_Count]  "<LSV_Vehicles_Count>"
  [LSV_Vehicles_Count] -> MATLAB Function/1(LSV_Vehicles_Count)
  [LSV_Elem1] -> Bus Selector41/1
  [Target_valid] -> Bus Selector47/1
  Bus Selector47/2 -> MATLAB Function/12(Target2_valid)  "<Target2_valid>"
  Bus Selector47/1 -> MATLAB Function/11(Target1_valid)  "<Target1_valid>"
  Bus Selector47/3 -> MATLAB Function/13(Target3_valid)  "<Target3_valid>"
  Bus Selector47/4 -> MATLAB Function/14(Target4_valid)  "<Target4_valid>"
  Bus Selector47/5 -> MATLAB Function/15(Target5_valid)  "<Target5_valid>"
  Bus Selector47/6 -> MATLAB Function/16(Target6_valid)  "<Target6_valid>"
  Unit Delay/1 -> MATLAB Function1/22(LSV_ListK)

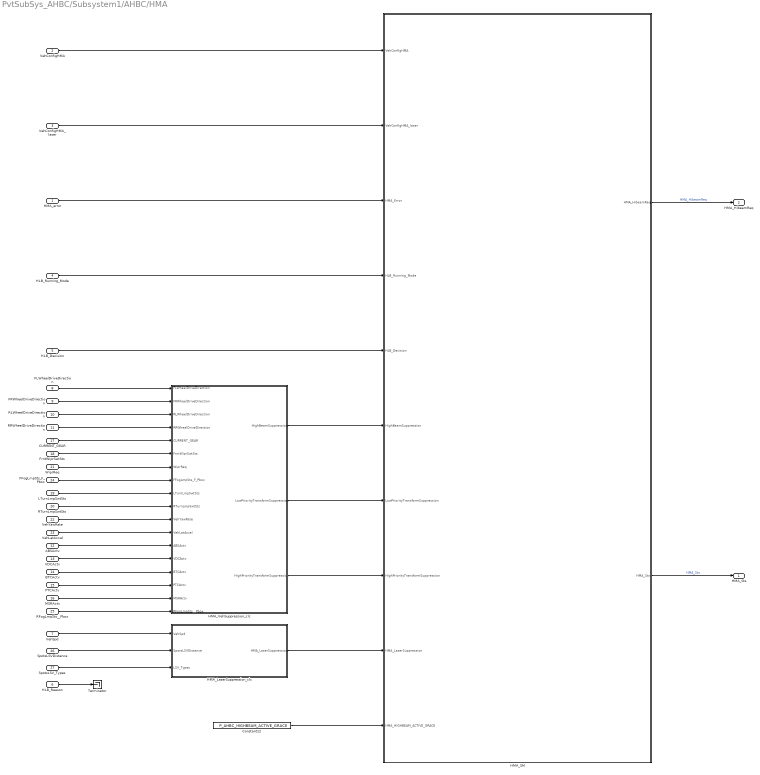
== system PvtSubSys_AHBC/Subsystem1/AHBC/HMA ==
  HMA_error : Inport
  VehConfigHMA : Inport  Port=2
  VehConfigHMA_laser : Inport  Port=3
  HLB_Running_Mode : Inport  Port=4
  HLB_Decision : Inport  Port=5
  HLB_Reason : Inport  Port=6
  VehSpd : Inport  Port=7
  FLWheelDriveDirection : Inport  Port=8
  FRWheelDriveDirection : Inport  Port=9
  RLWheelDriveDirection : Inport  Port=10
  RRWheelDriveDirection : Inport  Port=11
  ABSActv : Inport  Port=12
  VDCActv : Inport  Port=13
  BTCActv : Inport  Port=14
  PTCActv : Inport  Port=15
  MSRActv : Inport  Port=16
  CURRENT_GEAR : Inport  Port=17
  FrntWiprSwtSts : Inport  Port=18
  LTurnLmpSwtSts : Inport  Port=19
  RTurnLmpSwtSts : Inport  Port=20
  WiprReq : Inport  Port=21
  VehYawRate : Inport  Port=22
  VehLatAccel : Inport  Port=23
  FFogLmpSts_F_Pbox : Inport  Port=24
  RFogLmpSts__Pbox : Inport  Port=25
  SpotsLSVDistance : Inport  Port=26
  SpotsLSV_Types : Inport  Port=27
  Constant12 : Constant  Value=P_AHBC_HIGHBEAM_ACTIVE_GRACE
  HMA_LaserSuppression_clc : Subsystem
  HMA_SM : Stateflow chart  TreatAsAtomicUnit=on
  HMA_VehSuppression_clc : Subsystem
  Terminator : Terminator
  HMA_Sts : Outport  OutDataTypeStr=uint8
  HMA_HibeamReq : Outport  Port=2  OutDataTypeStr=uint8
  wires:
  RFogLmpSts__Pbox/1 -> HMA_VehSuppression_clc/18(RFogLmpSts__Pbox)
  HLB_Reason/1 -> Terminator/1
  HMA_SM/1(HMA_HibeamReq) -> HMA_HibeamReq/1  "HMA_HibeamReq"
  Constant12/1 -> HMA_SM/10(HMA_HIGHBEAM_ACTIVE_GRACE)
  CURRENT_GEAR/1 -> HMA_VehSuppression_clc/5(CURRENT_GEAR)
  RLWheelDriveDirection/1 -> HMA_VehSuppression_clc/3(RLWheelDriveDirection)
  FLWheelDriveDirection/1 -> HMA_VehSuppression_clc/1(FLWheelDriveDirection)
  HMA_error/1 -> HMA_SM/3(HMA_Error)
  WiprReq/1 -> HMA_VehSuppression_clc/7(WiprReq)
  VehYawRate/1 -> HMA_VehSuppression_clc/11(VehYawRate)
  BTCActv/1 -> HMA_VehSuppression_clc/15(BTCActv)
  FRWheelDriveDirection/1 -> HMA_VehSuppression_clc/2(FRWheelDriveDirection)
  SpotsLSVDistance/1 -> HMA_LaserSuppression_clc/2(SpotsLSVDistance)
  HMA_SM/2(HMA_Sts) -> HMA_Sts/1  "HMA_Sts"
  VehConfigHMA/1 -> HMA_SM/1(VehConfigHMA)
  HLB_Running_Mode/1 -> HMA_SM/4(HLB_Running_Mode)
  VehSpd/1 -> HMA_LaserSuppression_clc/1(VehSpd)
  VehConfigHMA_laser/1 -> HMA_SM/2(VehConfigHMA_laser)
  HLB_Decision/1 -> HMA_SM/5(HLB_Decision)
  FFogLmpSts_F_Pbox/1 -> HMA_VehSuppression_clc/8(FFogLmpSts_F_Pbox)
  SpotsLSV_Types/1 -> HMA_LaserSuppression_clc/3(LSV_Types)
  RRWheelDriveDirection/1 -> HMA_VehSuppression_clc/4(RRWheelDriveDirection)
  VehLatAccel/1 -> HMA_VehSuppression_clc/12(VehLatAccel)
  HMA_VehSuppression_clc/1(HighBeamSuppression) -> HMA_SM/6(HighBeamSuppression)
  RTurnLmpSwtSts/1 -> HMA_VehSuppression_clc/10(RTurnLmpSwtSts)
  HMA_VehSuppression_clc/3(HighPriorityTransformSuppression) -> HMA_SM/8(HighPriorityTransformSuppression)
  VDCActv/1 -> HMA_VehSuppression_clc/14(VDCActv)
  HMA_LaserSuppression_clc/1(HMA_LaserSuppression) -> HMA_SM/9(HMA_LaserSuppression)
  HMA_VehSuppression_clc/2(LowPriorityTransformSuppression) -> HMA_SM/7(LowPriorityTransformSuppression)
  LTurnLmpSwtSts/1 -> HMA_VehSuppression_clc/9(LTurnLmpSwtSts)
  ABSActv/1 -> HMA_VehSuppression_clc/13(ABSActv)
  PTCActv/1 -> HMA_VehSuppression_clc/16(PTCActv)
  MSRActv/1 -> HMA_VehSuppression_clc/17(MSRActv)
  FrntWiprSwtSts/1 -> HMA_VehSuppression_clc/6(FrntWiprSwtSts)
